simulink model "suspension_auto"  (R2022b)
settings: Solver=VariableStepAuto  StartTime=0.0  StopTime=10.0  MaxStep=0.00001  RelTol=1e-3
values from neighbouring files (symbols this model uses):
  b1 = 1000    [MOV_TRANS.m]    (also in datos_simulink.m)
  k1 = 16182    [MOV_TRANS.m]    (also in datos_simulink.m)
  k2 = 19000    [MOV_TRANS.m]    (also in datos_simulink.m)
  m1 = 290    [MOV_TRANS.m]    (also in datos_simulink.m)
  m2 = 59    [MOV_TRANS.m]    (also in datos_simulink.m)
  z = 0.05*sin(0.5*pi)    [MOV_TRANS.m]    (also in datos_simulink.m)
libraries: fl_lib x11, nesl_utility x4
settings Model: Creator=Cris  LastModifiedBy=Cris

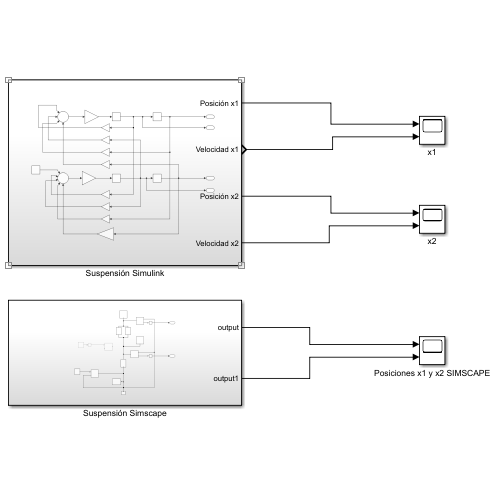
[thumbnail: Simulink's stored preview of the top-level diagram]
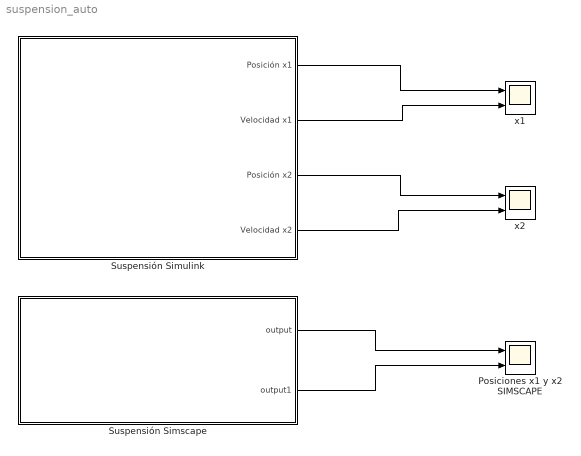
== system suspension_auto ==
  Posiciones x1 y x2 SIMSCAPE : Scope  NumInputPorts=2
  Suspensión Simscape : Subsystem
  Suspensión Simulink : Subsystem
  x1 : Scope  NumInputPorts=2
  x2 : Scope  NumInputPorts=2
  wires:
  Suspensión Simulink/1(Posición x1) -> x1/1
  Suspensión Simulink/2(Velocidad x1) -> x1/2
  Suspensión Simulink/3(Posición x2) -> x2/1
  Suspensión Simulink/4(Velocidad x2) -> x2/2
  Suspensión Simscape/1(output) -> Posiciones x1 y x2 SIMSCAPE/1
  Suspensión Simscape/2(output1) -> Posiciones x1 y x2 SIMSCAPE/2

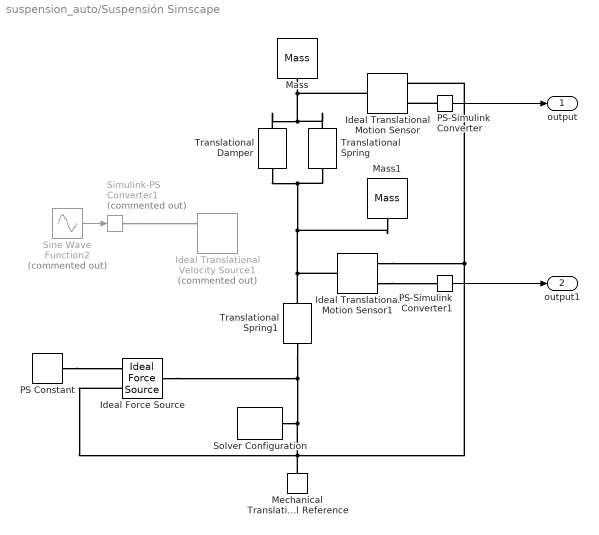
== system suspension_auto/Suspensión Simscape ==
  Ideal Force Source : fl_lib/Mechanical/Mechanical Sources/Ideal Force Source
  Ideal Translational Motion Sensor : fl_lib/Mechanical/Mechanical Sensors/Ideal Translational Motion Sensor  reference=foundation.enum.MeasurementReference.difference  acceleration_port=false  velocity_port=false  position_port=true  offset=0 m
      settings: InternalSimscapePortConfiguration="{\"Bottom\":[],\"Left\":[{\"id\":\"R\",\"label\":\"R\",\"type\":\"foundation.mechanical.translational.translational\"}],\"Right\":[{\"id\":\"C\",\"label\":\"C\",\"type\":\"foundation.mechanical.translational.translational\"},{\"id\":\"P\",\"label\":\"P\",\"type\":\"output\"}],\"Top\":[]}"
  Ideal Translational Motion Sensor1 : fl_lib/Mechanical/Mechanical Sensors/Ideal Translational Motion Sensor  reference=foundation.enum.MeasurementReference.difference  acceleration_port=false  velocity_port=false  position_port=true  offset=0 m
      settings: InternalSimscapePortConfiguration="{\"Bottom\":[],\"Left\":[{\"id\":\"R\",\"label\":\"R\",\"type\":\"foundation.mechanical.translational.translational\"}],\"Right\":[{\"id\":\"C\",\"label\":\"C\",\"type\":\"foundation.mechanical.translational.translational\"},{\"id\":\"P\",\"label\":\"P\",\"type\":\"output\"}],\"Top\":[]}"
  Ideal Translational Velocity Source1 : fl_lib/Mechanical/Mechanical Sources/Ideal Translational Velocity Source  Commented=on
  Mass : fl_lib/Mechanical/Translational Elements/Mass  mass=m1 kg  num_ports=foundation.enum.numPorts2.one  v_specify=off  v_priority=High  v=0 m/s  v_nominal_specify=off  v_nominal_unit=m/s  v_nominal_value=1  f_specify=off  f_priority=None  f=0 N  f_nominal_specify=off  f_nominal_unit=N  f_nominal_value=1
  Mass1 : fl_lib/Mechanical/Translational Elements/Mass  mass=m2 kg  num_ports=foundation.enum.numPorts2.one  v_specify=off  v_priority=High  v=0 m/s  v_nominal_specify=off  v_nominal_unit=m/s  v_nominal_value=1  f_specify=off  f_priority=None  f=0 N  f_nominal_specify=off  f_nominal_unit=N  f_nominal_value=1
  Mechanical Translational Reference : fl_lib/Mechanical/Translational Elements/Mechanical Translational Reference
  PS Constant : fl_lib/Physical Signals/Sources/PS Constant  constant=0
  PS-Simulink Converter : nesl_utility/PS-Simulink Converter  PhysicalDomain=network_engine_domain  SubClassName=ps_output  LeftPortType=input  RightPortType=output  PseudoPeriodic=off  Frequencies=[]  VectorFormat=inherit  Unit=inherit  AffineConversion=off
  PS-Simulink Converter1 : nesl_utility/PS-Simulink Converter  PhysicalDomain=network_engine_domain  SubClassName=ps_output  LeftPortType=input  RightPortType=output  PseudoPeriodic=off  Frequencies=[]  VectorFormat=inherit  Unit=inherit  AffineConversion=off
  Simulink-PS Converter1 : nesl_utility/Simulink-PS Converter  Commented=on  PhysicalDomain=network_engine_domain  SubClassName=ps_input  LeftPortType=input  RightPortType=output  PseudoPeriodic=off  Frequencies=[]  NoiseDistribution=none  NoiseParameters=[]  Unit=1  AffineConversion=off  FilteringAndDerivatives=provide  SimscapeFilterOrder=1  InputFilterTimeConstant=0.001  UdotUserProvided=0
  Sine Wave Function2 : Sin  Commented=on  Amplitude=0.05*k2  Frequency=62.83  SampleTime=0
  Solver Configuration : nesl_utility/Solver Configuration  PhysicalDomain=network_engine_domain  SubClassName=solver  LeftPortType=input  RightPortType=generic  Tones=[]  Harmonics=[]  SimulateNoise=off  Profile=off  UseLocalSampling=off  EnableSwitchedLinearOptims=on  FrequencyDomain=off  UseCCode=off  RelTol=0.001  AbsTol=0.001  MinStep=1e-09  ToWorkspace=off  RevertToSquareIcSolve=off  NumHomotopyIterations=100  PhasorMode=off  PhasorModeNumHarmonics=1  ConsistencySolver=NEWTON_XTOL_AFTER_FTOL  IndexReductionMethod=DerivativeReplacement  DoDC=off  ResidualTolerance=1e-09  ConsistencyTolSource=GLOBAL  ConsistencyAbsTol=0.001  ConsistencyRelTol=0.001  ConsistencyTolFactor=0.001  UseLocalSolver=off  LocalSolverChoice=NE_BACKWARD_EULER_ADVANCER  ResolveIndetEquations=on  FunctionEvalNumThread=1  LocalSolverSampleTime=0.001  DoFixedCost=off  MaxNonlinIter=3  MaxModeIter=2  ComputeImpulses=off  ImpulseIterations=2  LinearAlgebra=auto  LinearAlgebraNumThread=0  EquationFormulation=NE_TIME_EF  DelaysMemoryBudget=1024  AutomaticFiltering=on  FilteringTimeConstant=0.001  PartitionStorageMethod=AS_NEEDED  PartitionMemoryBudget=1024  PartitionMethod=ROBUST
  Translational Damper : fl_lib/Mechanical/Translational Elements/Translational Damper  D=b1 N*s/m  v_specify=off  v_priority=None  v=0 m/s  v_nominal_specify=off  v_nominal_unit=m/s  v_nominal_value=1  f_specify=off  f_priority=None  f=0 N  f_nominal_specify=off  f_nominal_unit=N  f_nominal_value=1
  Translational Spring : fl_lib/Mechanical/Translational Elements/Translational Spring  spr_rate=k1 N/m  v_specify=off  v_priority=None  v=0 m/s  v_nominal_specify=off  v_nominal_unit=m/s  v_nominal_value=1  f_specify=off  f_priority=None  f=0 N  f_nominal_specify=off  f_nominal_unit=N  f_nominal_value=1  x_specify=off  x_priority=High  x=0 m  x_nominal_specify=off  x_nominal_unit=m  x_nominal_value=1
  Translational Spring1 : fl_lib/Mechanical/Translational Elements/Translational Spring  spr_rate=k2 N/m  v_specify=off  v_priority=None  v=0 m/s  v_nominal_specify=off  v_nominal_unit=m/s  v_nominal_value=1  f_specify=off  f_priority=None  f=0 N  f_nominal_specify=off  f_nominal_unit=N  f_nominal_value=1  x_specify=on  x_priority=High  x=z m  x_nominal_specify=off  x_nominal_unit=m  x_nominal_value=1
  output : Outport
  output1 : Outport  Port=2
  wires:
  PS-Simulink Converter/1 -> output/1
  PS-Simulink Converter1/1 -> output1/1
  Sine Wave Function2/1 -> Simulink-PS Converter1/1
  connections:
  PS-Simulink Converter/LConn1 -- Ideal Translational Motion Sensor/RConn2
  Solver Configuration/RConn1 -- Translational Spring1/LConn1 -- Ideal Force Source/LConn1 -- Ideal Translational Motion Sensor1/RConn1 -- Ideal Translational Motion Sensor/RConn1 -- Ideal Force Source/RConn2 -- Mechanical Translational Reference/LConn1
  Mass1/LConn1 -- Translational Spring1/RConn1 -- Ideal Translational Motion Sensor1/LConn1 -- Translational Spring/LConn1 -- Translational Damper/LConn1
  Ideal Translational Motion Sensor/LConn1 -- Translational Spring/RConn1 -- Translational Damper/RConn1 -- Mass/LConn1
  Ideal Translational Motion Sensor1/RConn2 -- PS-Simulink Converter1/LConn1
  Simulink-PS Converter1/RConn1 -- Ideal Translational Velocity Source1/RConn1
  PS Constant/RConn1 -- Ideal Force Source/RConn1

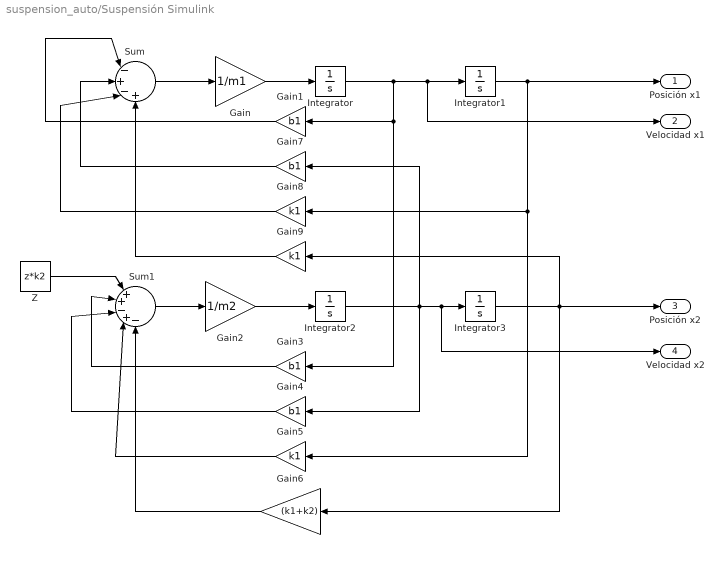
== system suspension_auto/Suspensión Simulink ==
  Gain : Gain  Gain=1/m1
  Gain{1,3..4,7} (4 alike) : Gain  Gain=b1
  Gain2 : Gain  Gain=1/m2
  Gain5 : Gain  Gain=k1
  Gain6 : Gain  Gain=(k1+k2)
  Gain8 : Gain  Gain=k1
  Gain9 : Gain  Gain=k1
  Integrator{,1..3} (4 alike) : Integrator
  Sum : Sum  Inputs=|-+-+
  Sum1 : Sum  Inputs=|++-+-
  Z : Constant  Value=z*k2
  Posición x1 : Outport
  Velocidad x1 : Outport  Port=2
  Posición x2 : Outport  Port=3
  Velocidad x2 : Outport  Port=4
  wires:
  Integrator/1 -> Gain3/1, Gain1/1, Velocidad x1/1, Integrator1/1
  Integrator2/1 -> Gain4/1, Gain7/1, Velocidad x2/1, Integrator3/1
  Sum/1 -> Gain/1
  Gain1/1 -> Sum/1
  Sum1/1 -> Gain2/1
  Gain5/1 -> Sum1/4
  Integrator3/1 -> Posición x2/1, Gain9/1, Gain6/1
  Integrator1/1 -> Posición x1/1, Gain8/1, Gain5/1
  Gain2/1 -> Integrator2/1
  Gain9/1 -> Sum/4
  Gain7/1 -> Sum/2
  Gain3/1 -> Sum1/2
  Gain4/1 -> Sum1/3
  Gain6/1 -> Sum1/5
  Gain8/1 -> Sum/3
  Z/1 -> Sum1/1
  Gain/1 -> Integrator/1
